simulink model "s_sip_freefall_ss_vs_eom"  (Simulink 4.00)
settings: Solver=ode4  SolverMode=SingleTasking  StartTime=0.0  StopTime=3  FixedStep=0.001  RelTol=1e-3  AbsTol=1e-6
values from neighbouring files (symbols this model uses):
  Bp = 0.0024    [setup_sp_configuration.m]
  g = 9.81    [setup_sp_configuration.m]
  IC_ALPHA0 = IC_ALPHA0 / 180 * pi    (= 0)    [setup_lab_ip01_2_sip.m]
  Ip = Mp * Lp^2 / 12    [setup_sp_configuration.m]
  lp = 7 * K_IN2M    [setup_sp_configuration.m]
  Mc = Mc + Eff_g * Kg^2 * Jm / r_mp^2    [setup_lab_ip01_2_sip.m]
  Mp = 0.127    [setup_sp_configuration.m]
undefined symbols (not defined in the file or in its folder): A, B, Beq, C, D, Eff_g, Eff_m, IMAX_UPM, Kg, Km, Kt, r_mp, Rm
libraries: simulink_extras x1
settings Model: LastModifiedBy=herve  LimitDataPoints=off  RTWSystemTargetFile=wincon.tlc  RTWTemplateMakefile=nt_msvc.tmf  RTWMakeCommand=make_wc  ExtModeMexFile=wc_comm  ExtModeArmWhenConnect=off  OptimizeBlockIOStorage=off

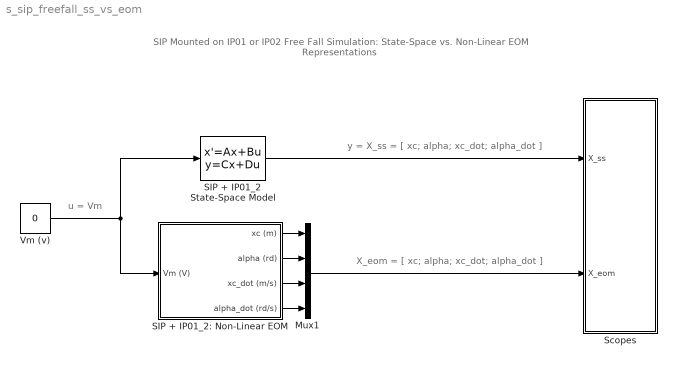
== system s_sip_freefall_ss_vs_eom ==
  note: SIP Mounted on IP01 or IP02
      | Free Fall Simulation:
      | State-Space vs. Non-Linear EOM Representations
  note: u = Vm
  note: y = X_ss = [ xc; alpha; xc_dot; alpha_dot ]
  note: X_eom = [ xc; alpha; xc_dot; alpha_dot ]
  Mux1 : Mux  Inputs=4
  SIP + IP01_2 State-Space Model : StateSpace  A=A  B=B  C=C  D=D  X0=[ 0; IC_ALPHA0; 0; 0 ]  AbsoluteTolerance=auto  Realization=auto
  SIP + IP01_2: Non-Linear EOM : Subsystem
      settings: RTWFcnNameOpts=Auto  RTWFileNameOpts=Auto
  Scopes : Subsystem
      settings: RTWFcnNameOpts=Auto  RTWFileNameOpts=Auto
  Vm (v) : Constant  Value=0
  wires:
  Vm (v)/1 -> SIP + IP01_2 State-Space Model/1, SIP + IP01_2: Non-Linear EOM/1(Vm (V))
  Mux1/1 -> Scopes/2(X_eom)
  SIP + IP01_2 State-Space Model/1 -> Scopes/1(X_ss)
  SIP + IP01_2: Non-Linear EOM/1(xc (m)) -> Mux1/1
  SIP + IP01_2: Non-Linear EOM/2(alpha (rd)) -> Mux1/2
  SIP + IP01_2: Non-Linear EOM/3(xc_dot (m/s)) -> Mux1/3
  SIP + IP01_2: Non-Linear EOM/4(alpha_dot (rd/s)) -> Mux1/4

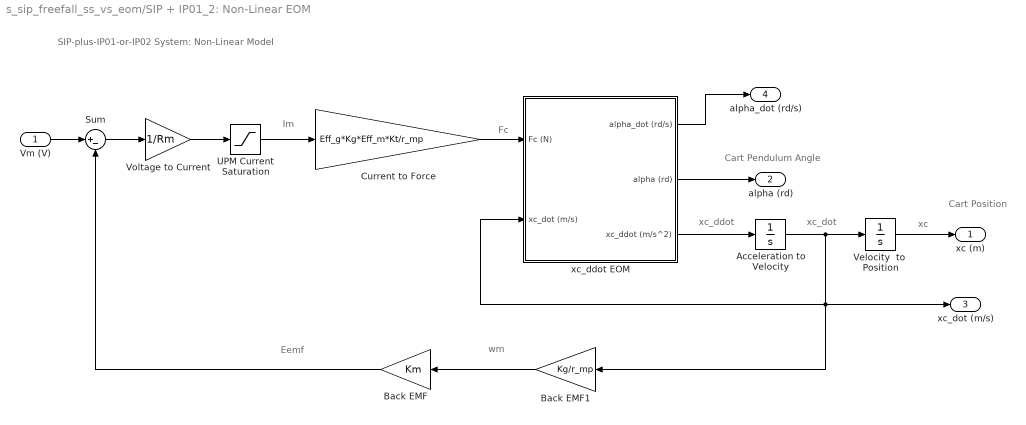
== system s_sip_freefall_ss_vs_eom/SIP + IP01_2: Non-Linear EOM ==
  note: SIP-plus-IP01-or-IP02 System:
      | Non-Linear Model
  note: Fc
  note: Im
  note: Eemf
  note: wm
  note: xc_dot
  note: xc_ddot
  note: xc
  note: Cart Position
  note: Cart Pendulum Angle
  Vm (V) : Inport  Port=1  LatchInput=off
  Acceleration to Velocity : Integrator  ExternalReset=none  InitialConditionSource=internal  InitialCondition=0  LimitOutput=off  UpperSaturationLimit=inf  LowerSaturationLimit=-inf  ShowSaturationPort=off  ShowStatePort=off  AbsoluteTolerance=auto
  Back EMF : Gain  Orientation=left  Gain=Km  Multiplication=Element-wise(K.*u)  SaturateOnIntegerOverflow=on
  Back EMF1 : Gain  Orientation=left  Gain=Kg/r_mp  Multiplication=Element-wise(K.*u)  SaturateOnIntegerOverflow=on
  Current to Force : Gain  Gain=Eff_g*Kg*Eff_m*Kt/r_mp  Multiplication=Element-wise(K.*u)  SaturateOnIntegerOverflow=on
  Sum : Sum  Inputs=|+-  SaturateOnIntegerOverflow=on
  "UPM Current Saturation " : Saturate  UpperLimit=IMAX_UPM  LowerLimit=- IMAX_UPM  LinearizeAsGain=on
  Velocity  to  Position : Integrator  ExternalReset=none  InitialConditionSource=internal  InitialCondition=0  LimitOutput=off  UpperSaturationLimit=inf  LowerSaturationLimit=-inf  ShowSaturationPort=off  ShowStatePort=off  AbsoluteTolerance=auto
  Voltage to Current : Gain  Gain=1/Rm  Multiplication=Element-wise(K.*u)  SaturateOnIntegerOverflow=on
  xc_ddot EOM : Subsystem
      settings: RTWFcnNameOpts=Auto  RTWFileNameOpts=Auto
  xc (m) : Outport  Port=1
  alpha (rd) : Outport  Port=2
  xc_dot (m/s) : Outport  Port=3  InitialOutput=0
  alpha_dot (rd/s) : Outport  Port=4  InitialOutput=0
  wires:
  Sum/1 -> Voltage to Current/1
  Voltage to Current/1 -> "UPM Current Saturation "/1
  Acceleration to Velocity/1 -> xc_dot (m/s)/1, xc_ddot EOM/2(xc_dot (m/s)), Back EMF1/1, Velocity  to  Position/1
  Back EMF1/1 -> Back EMF/1
  Vm (V)/1 -> Sum/1
  Velocity  to  Position/1 -> xc (m)/1
  Back EMF/1 -> Sum/2
  "UPM Current Saturation "/1 -> Current to Force/1
  Current to Force/1 -> xc_ddot EOM/1(Fc (N))
  xc_ddot EOM/3(xc_ddot (m/s^2)) -> Acceleration to Velocity/1
  xc_ddot EOM/1(alpha_dot (rd/s)) -> alpha_dot (rd/s)/1
  xc_ddot EOM/2(alpha (rd)) -> alpha (rd)/1

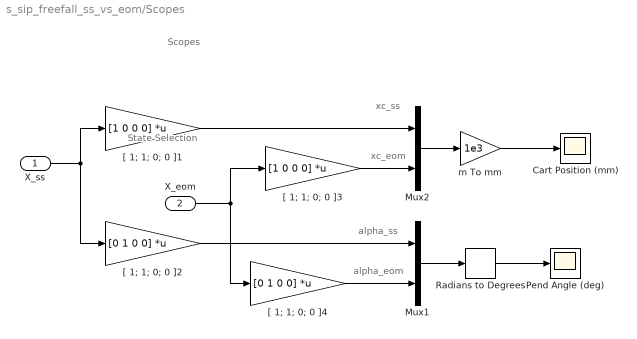
== system s_sip_freefall_ss_vs_eom/Scopes ==
  note: xc_ss
  note: State Selection
  note: alpha_ss
  note: alpha_eom
  note: xc_eom
  note: Scopes
  X_ss : Inport  Port=1  LatchInput=off
  X_eom : Inport  Port=2  LatchInput=off
  Cart Position (mm) : Scope
      settings: TickLabels=on  TimeRange=3  YMin=-50  YMax=50  SaveToWorkspace=off  DataFormat=Array  LimitDataPoints=on  MaxDataPoints=5000
  Mux1 : Mux  Inputs=2
  Mux2 : Mux  Inputs=2
  Pend Angle (deg) : Scope
      settings: TickLabels=on  TimeRange=3  YMin=-2  YMax=320  SaveToWorkspace=off  SaveName=ScopeData  DataFormat=Array  LimitDataPoints=on  MaxDataPoints=5000
  Radians to Degrees : simulink_extras/Transformations/Radians to Degrees
  "[ 1; 1; 0; 0 ]1" : Gain  Gain=[1 0 0 0]  Multiplication=Matrix(K*u)  SaturateOnIntegerOverflow=on
  "[ 1; 1; 0; 0 ]2" : Gain  Gain=[0 1 0 0]  Multiplication=Matrix(K*u)  SaturateOnIntegerOverflow=on
  "[ 1; 1; 0; 0 ]3" : Gain  Gain=[1 0 0 0]  Multiplication=Matrix(K*u)  SaturateOnIntegerOverflow=on
  "[ 1; 1; 0; 0 ]4" : Gain  Gain=[0 1 0 0]  Multiplication=Matrix(K*u)  SaturateOnIntegerOverflow=on
  m To mm : Gain  Gain=1e3  Multiplication=Element-wise(K.*u)  SaturateOnIntegerOverflow=on
  wires:
  Mux2/1 -> m To mm/1
  m To mm/1 -> Cart Position (mm)/1
  X_ss/1 -> "[ 1; 1; 0; 0 ]1"/1, "[ 1; 1; 0; 0 ]2"/1
  Mux1/1 -> Radians to Degrees/1
  Radians to Degrees/1 -> Pend Angle (deg)/1
  X_eom/1 -> "[ 1; 1; 0; 0 ]3"/1, "[ 1; 1; 0; 0 ]4"/1
  "[ 1; 1; 0; 0 ]3"/1 -> Mux2/2
  "[ 1; 1; 0; 0 ]4"/1 -> Mux1/2
  "[ 1; 1; 0; 0 ]2"/1 -> Mux1/1
  "[ 1; 1; 0; 0 ]1"/1 -> Mux2/1

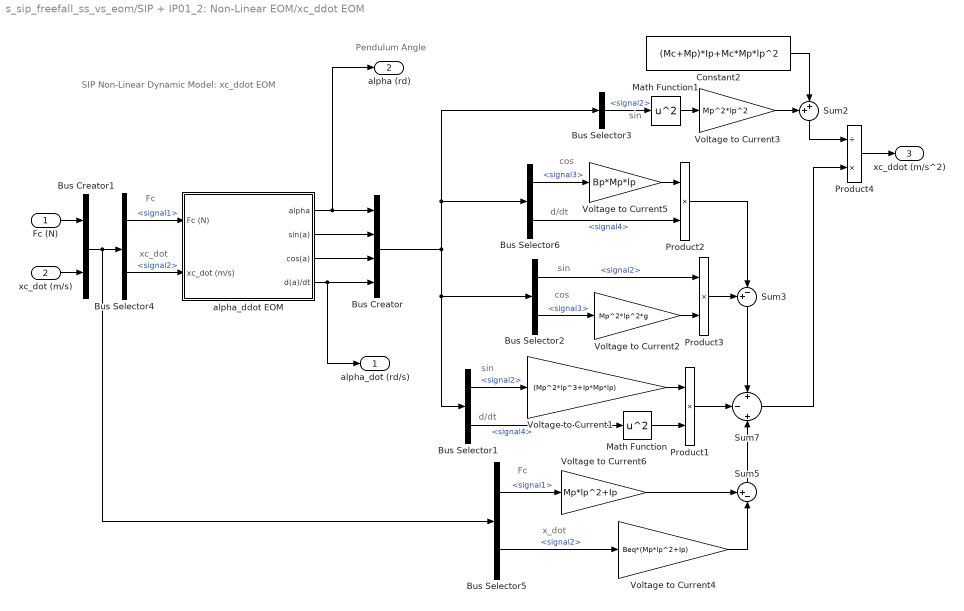
== system s_sip_freefall_ss_vs_eom/SIP + IP01_2: Non-Linear EOM/xc_ddot EOM ==
  note: xc_dot
  note: Fc
  note: x_dot
  note: Fc
  note: d/dt
  note: cos
  note: Pendulum Angle
  note: sin
  note: cos
  note: sin
  note: sin
  note: d/dt
  note: SIP Non-Linear Dynamic Model:
      | xc_ddot EOM
  Fc (N) : Inport  Port=1  LatchInput=off
  xc_dot (m/s) : Inport  Port=2  LatchInput=off
  Bus Creator : BusCreator  Inputs=4
  Bus Creator1 : BusCreator  Inputs=2
  Bus Selector1 : BusSelector  OutputSignals=signal2,signal4  MuxedOutput=off
  Bus Selector2 : BusSelector  OutputSignals=signal2,signal3  MuxedOutput=off
  Bus Selector3 : BusSelector  OutputSignals=signal2  MuxedOutput=off
  Bus Selector4 : BusSelector  OutputSignals=signal1,signal2  MuxedOutput=off
  Bus Selector5 : BusSelector  OutputSignals=signal1,signal2  MuxedOutput=off
  Bus Selector6 : BusSelector  OutputSignals=signal3,signal4  MuxedOutput=off
  Constant2 : Constant  Value=(Mc+Mp)*Ip+Mc*Mp*lp^2
  Math Function : Math  Operator=square  OutputSignalType=auto
  Math Function1 : Math  Operator=square  OutputSignalType=auto
  Product1 : Product  Inputs=2  Multiplication=Element-wise(.*)  SaturateOnIntegerOverflow=on
  Product2 : Product  Inputs=2  Multiplication=Element-wise(.*)  SaturateOnIntegerOverflow=on
  Product3 : Product  Inputs=2  Multiplication=Element-wise(.*)  SaturateOnIntegerOverflow=on
  Product4 : Product  Inputs=/*  Multiplication=Element-wise(.*)  SaturateOnIntegerOverflow=on
  Sum2 : Sum  Orientation=down  Inputs=++|  SaturateOnIntegerOverflow=on
  Sum3 : Sum  Orientation=down  Inputs=+-|  SaturateOnIntegerOverflow=on
  Sum5 : Sum  Orientation=up  Inputs=+-|  SaturateOnIntegerOverflow=on
  Sum7 : Sum  Inputs=+|-|+  SaturateOnIntegerOverflow=on
  Voltage to Current1 : Gain  Gain=(Mp^2*lp^3+Ip*Mp*lp)  Multiplication=Element-wise(K.*u)  SaturateOnIntegerOverflow=on
  Voltage to Current2 : Gain  Gain=Mp^2*lp^2*g  Multiplication=Element-wise(K.*u)  SaturateOnIntegerOverflow=on
  Voltage to Current3 : Gain  Gain=Mp^2*lp^2  Multiplication=Element-wise(K.*u)  SaturateOnIntegerOverflow=on
  Voltage to Current4 : Gain  Gain=Beq*(Mp*lp^2+Ip)  Multiplication=Element-wise(K.*u)  SaturateOnIntegerOverflow=on
  Voltage to Current5 : Gain  Gain=Bp*Mp*lp  Multiplication=Element-wise(K.*u)  SaturateOnIntegerOverflow=on
  Voltage to Current6 : Gain  Gain=Mp*lp^2+Ip  Multiplication=Element-wise(K.*u)  SaturateOnIntegerOverflow=on
  alpha_ddot EOM : Subsystem
      settings: RTWFcnNameOpts=Auto  RTWFileNameOpts=Auto
  alpha_dot (rd/s) : Outport  Port=1
  alpha (rd) : Outport  Port=2
  xc_ddot (m/s^2) : Outport  Port=3
  wires:
  Voltage to Current4/1 -> Sum5/2
  Voltage to Current6/1 -> Sum5/1
  Sum5/1 -> Sum7/3
  Sum3/1 -> Sum7/1
  Product3/1 -> Sum3/1
  Product2/1 -> Sum3/2
  Sum7/1 -> Product4/2
  Bus Selector5/2 -> Voltage to Current4/1  "<signal2>"
  Bus Selector5/1 -> Voltage to Current6/1  "<signal1>"
  Voltage to Current5/1 -> Product2/1
  Bus Selector2/2 -> Voltage to Current2/1  "<signal3>"
  Bus Selector2/1 -> Product3/1  "<signal2>"
  Bus Selector6/2 -> Product2/2  "<signal4>"
  Bus Selector6/1 -> Voltage to Current5/1  "<signal3>"
  Bus Selector1/1 -> Voltage to Current1/1  "<signal2>"
  Bus Selector1/2 -> Math Function/1  "<signal4>"
  Bus Selector4/2 -> alpha_ddot EOM/2(xc_dot (m/s))  "<signal2>"
  Bus Selector4/1 -> alpha_ddot EOM/1(Fc (N))  "<signal1>"
  Bus Creator1/1 -> Bus Selector5/1, Bus Selector4/1
  xc_dot (m/s)/1 -> Bus Creator1/2
  Fc (N)/1 -> Bus Creator1/1
  alpha_ddot EOM/4(d(a)/dt) -> Bus Creator/4, alpha_dot (rd/s)/1
  alpha_ddot EOM/3(cos(a)) -> Bus Creator/3
  alpha_ddot EOM/2(sin(a)) -> Bus Creator/2
  alpha_ddot EOM/1(alpha) -> alpha (rd)/1, Bus Creator/1
  Product4/1 -> xc_ddot (m/s^2)/1
  Product1/1 -> Sum7/2
  Constant2/1 -> Sum2/2
  Voltage to Current3/1 -> Sum2/1
  Math Function1/1 -> Voltage to Current3/1
  Bus Selector3/1 -> Math Function1/1  "<signal2>"
  Voltage to Current2/1 -> Product3/2
  Math Function/1 -> Product1/2
  Voltage to Current1/1 -> Product1/1
  Bus Creator/1 -> Bus Selector6/1, Bus Selector3/1, Bus Selector1/1, Bus Selector2/1
  Sum2/1 -> Product4/1

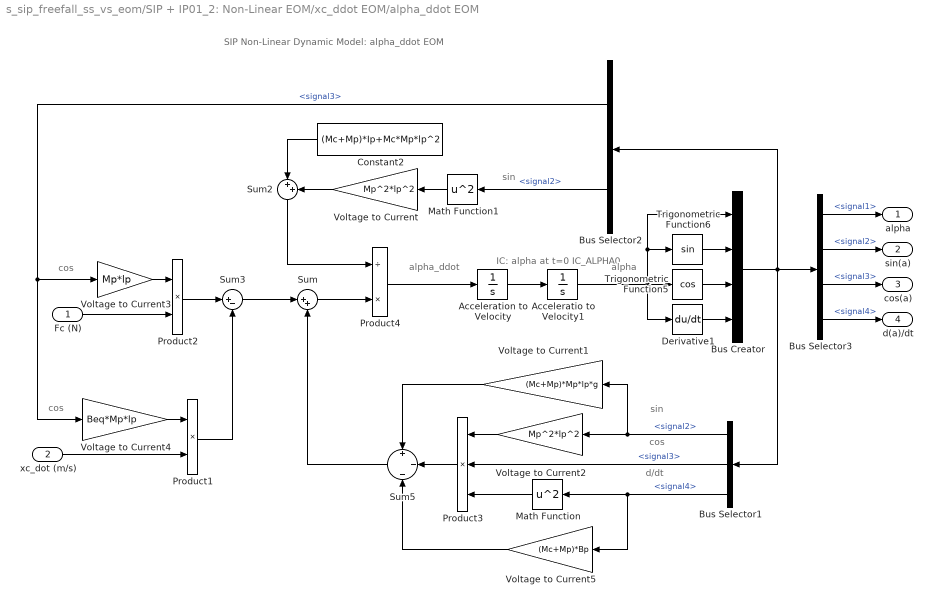
== system s_sip_freefall_ss_vs_eom/SIP + IP01_2: Non-Linear EOM/xc_ddot EOM/alpha_ddot EOM ==
  note: cos
  note: alpha_ddot
  note: IC: alpha at t=0
      | IC_ALPHA0
  note: SIP Non-Linear Dynamic Model:
      | alpha_ddot EOM
  note: alpha
  note: sin
  note: cos
  note: sin
  note: cos
  note: d/dt
  Fc (N) : Inport  Port=1  LatchInput=off
  xc_dot (m/s) : Inport  Port=2  LatchInput=off
  Acceleratio to Velocity1 : Integrator  ExternalReset=none  InitialConditionSource=internal  InitialCondition=IC_ALPHA0  LimitOutput=off  UpperSaturationLimit=inf  LowerSaturationLimit=-inf  ShowSaturationPort=off  ShowStatePort=off  AbsoluteTolerance=auto
  Acceleration to Velocity : Integrator  ExternalReset=none  InitialConditionSource=internal  InitialCondition=0  LimitOutput=off  UpperSaturationLimit=inf  LowerSaturationLimit=-inf  ShowSaturationPort=off  ShowStatePort=off  AbsoluteTolerance=auto
  Bus Creator : BusCreator  Inputs=4
  Bus Selector1 : BusSelector  Orientation=left  OutputSignals=signal2,signal3,signal4  MuxedOutput=off
  Bus Selector2 : BusSelector  Orientation=left  OutputSignals=signal3,signal2  MuxedOutput=off
  Bus Selector3 : BusSelector  OutputSignals=signal1,signal2,signal3,signal4  MuxedOutput=off
  Constant2 : Constant  Orientation=left  Value=(Mc+Mp)*Ip+Mc*Mp*lp^2
  Derivative1 : Derivative
  Math Function : Math  Orientation=left  Operator=square  OutputSignalType=auto
  Math Function1 : Math  Orientation=left  Operator=square  OutputSignalType=auto
  Product1 : Product  Inputs=2  Multiplication=Element-wise(.*)  SaturateOnIntegerOverflow=on
  Product2 : Product  Inputs=2  Multiplication=Element-wise(.*)  SaturateOnIntegerOverflow=on
  Product3 : Product  Orientation=left  Inputs=3  Multiplication=Element-wise(.*)  SaturateOnIntegerOverflow=on
  Product4 : Product  Inputs=/*  Multiplication=Element-wise(.*)  SaturateOnIntegerOverflow=on
  Sum : Sum  Inputs=|++  SaturateOnIntegerOverflow=on
  Sum2 : Sum  Orientation=down  Inputs=|++  SaturateOnIntegerOverflow=on
  Sum3 : Sum  Inputs=|+-  SaturateOnIntegerOverflow=on
  Sum5 : Sum  Orientation=left  Inputs=+|-|-  SaturateOnIntegerOverflow=on
  Trigonometric Function5 : Trigonometry  Operator=cos  OutputSignalType=auto
  Trigonometric Function6 : Trigonometry  Operator=sin  OutputSignalType=auto
  Voltage to Current : Gain  Orientation=left  Gain=Mp^2*lp^2  Multiplication=Element-wise(K.*u)  SaturateOnIntegerOverflow=on
  Voltage to Current1 : Gain  Orientation=left  Gain=(Mc+Mp)*Mp*lp*g  Multiplication=Element-wise(K.*u)  SaturateOnIntegerOverflow=on
  Voltage to Current2 : Gain  Orientation=left  Gain=Mp^2*lp^2  Multiplication=Element-wise(K.*u)  SaturateOnIntegerOverflow=on
  Voltage to Current3 : Gain  Gain=Mp*lp  Multiplication=Element-wise(K.*u)  SaturateOnIntegerOverflow=on
  Voltage to Current4 : Gain  Gain=Beq*Mp*lp  Multiplication=Element-wise(K.*u)  SaturateOnIntegerOverflow=on
  Voltage to Current5 : Gain  Orientation=left  Gain=(Mc+Mp)*Bp  Multiplication=Element-wise(K.*u)  SaturateOnIntegerOverflow=on
  alpha : Outport  Port=1  InitialOutput=0
  sin(a) : Outport  Port=2  InitialOutput=0
  cos(a) : Outport  Port=3  InitialOutput=0
  d(a)/dt : Outport  Port=4  InitialOutput=0
  wires:
  Sum5/1 -> Sum/2
  Voltage to Current5/1 -> Sum5/3
  Voltage to Current1/1 -> Sum5/1
  Product3/1 -> Sum5/2
  Sum3/1 -> Sum/1
  Product1/1 -> Sum3/2
  Product2/1 -> Sum3/1
  Voltage to Current4/1 -> Product1/1
  xc_dot (m/s)/1 -> Product1/2
  Fc (N)/1 -> Product2/2
  Voltage to Current3/1 -> Product2/1
  Acceleratio to Velocity1/1 -> Bus Creator/1, Trigonometric Function6/1, Derivative1/1, Trigonometric Function5/1
  Bus Selector3/4 -> d(a)/dt/1  "<signal4>"
  Bus Selector3/3 -> cos(a)/1  "<signal3>"
  Bus Selector3/2 -> sin(a)/1  "<signal2>"
  Bus Selector3/1 -> alpha/1  "<signal1>"
  Bus Selector1/3 -> Voltage to Current5/1, Math Function/1  "<signal4>"
  Bus Selector1/2 -> Product3/2  "<signal3>"
  Voltage to Current2/1 -> Product3/1
  Bus Selector2/1 -> Voltage to Current4/1, Voltage to Current3/1  "<signal3>"
  Bus Creator/1 -> Bus Selector3/1, Bus Selector1/1, Bus Selector2/1
  Derivative1/1 -> Bus Creator/4
  Trigonometric Function5/1 -> Bus Creator/3
  Trigonometric Function6/1 -> Bus Creator/2
  Constant2/1 -> Sum2/1
  Math Function1/1 -> Voltage to Current/1
  Bus Selector2/2 -> Math Function1/1  "<signal2>"
  Voltage to Current/1 -> Sum2/2
  Sum/1 -> Product4/2
  Sum2/1 -> Product4/1
  Math Function/1 -> Product3/3
  Product4/1 -> Acceleration to Velocity/1
  Bus Selector1/1 -> Voltage to Current2/1, Voltage to Current1/1  "<signal2>"
  Acceleration to Velocity/1 -> Acceleratio to Velocity1/1
